simulink model "calibration_sensors"  (R2026a)
settings: Solver=VariableStepAuto  StopTime=inf
StopFcn:
  | coefficients = out.coefficients;
  | sensor_low = out.sensor_low;
  | sensor_high = out.sensor_high;
  | 
  | save('sensor_calibration.mat', ...
  |      'coefficients', ...
  |      'sensor_low', ...
  |      'sensor_high');
(part 1 of 3)
settings Model: Creator=user  LastModifiedBy=jinyu

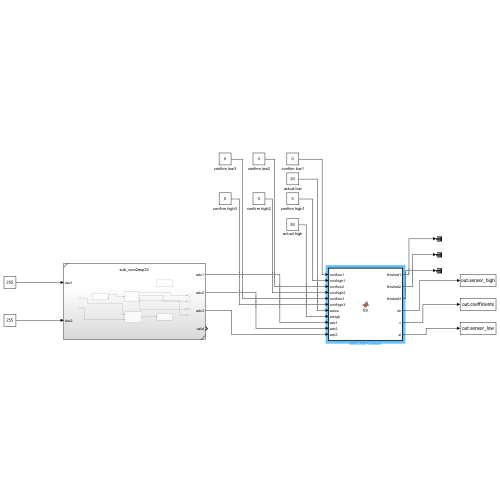
[thumbnail: Simulink's stored preview of the top-level diagram]
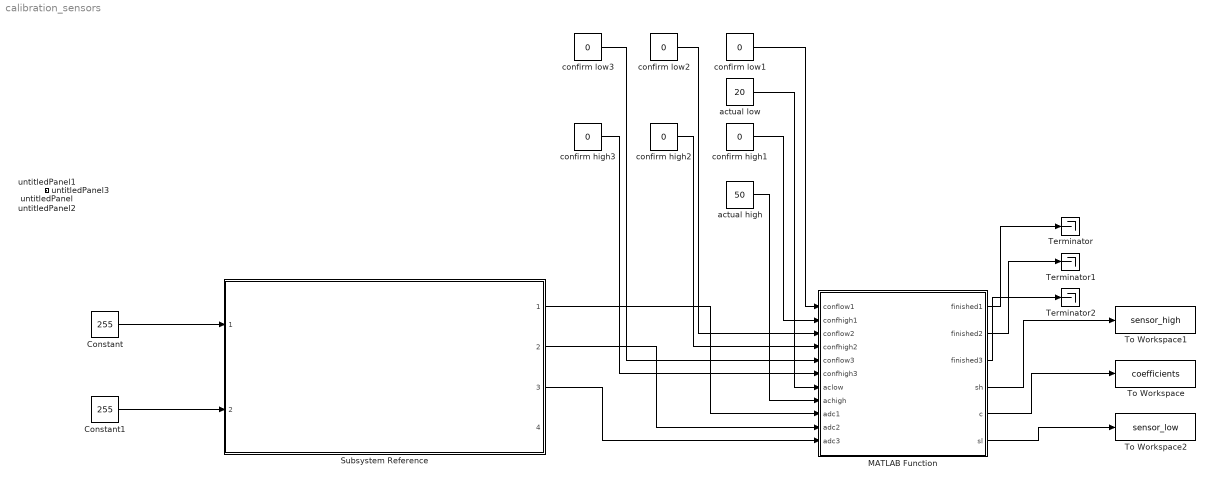
== system calibration_sensors ==
  Constant : Constant  Value=255
  Constant1 : Constant  Value=255
  MATLAB Function : MATLAB Function  TreatAsAtomicUnit=on
  Subsystem Reference : Subsystem  ReferencedSubsystem=sub_com2esp32
  Terminator : Terminator
  Terminator1 : Terminator
  Terminator2 : Terminator
  To Workspace : ToWorkspace  VariableName=coefficients  SampleTime=-1
      settings: MaxDataPoints=1
  To Workspace1 : ToWorkspace  VariableName=sensor_high  SampleTime=-1
      settings: MaxDataPoints=1
  To Workspace2 : ToWorkspace  VariableName=sensor_low  SampleTime=-1
      settings: MaxDataPoints=1
  actual high : Constant  Value=50
  actual low : Constant  Value=20
  confirm high1 : Constant  Value=0
  confirm high2 : Constant  Value=0
  confirm high3 : Constant  Value=0
  confirm low1 : Constant  Value=0
  confirm low2 : Constant  Value=0
  confirm low3 : Constant  Value=0
  untitledPanel : Subsystem  Tag=HiddenForWebPanel  IsWebBlockPanel=on
  untitledPanel1 : Subsystem  Tag=HiddenForWebPanel  IsWebBlockPanel=on
  untitledPanel2 : Subsystem  Tag=HiddenForWebPanel  IsWebBlockPanel=on
  untitledPanel3 : Subsystem  Tag=HiddenForWebPanel  IsWebBlockPanel=on
  wires:
  Constant/1 -> Subsystem Reference/1
  Constant1/1 -> Subsystem Reference/2
  Subsystem Reference/3 -> MATLAB Function/11(adc3)
  Subsystem Reference/1 -> MATLAB Function/9(adc1)
  Subsystem Reference/2 -> MATLAB Function/10(adc2)
  actual high/1 -> MATLAB Function/8(achigh)
  confirm high1/1 -> MATLAB Function/2(confhigh1)
  actual low/1 -> MATLAB Function/7(aclow)
  confirm low1/1 -> MATLAB Function/1(conflow1)
  MATLAB Function/5(c) -> To Workspace/1
  MATLAB Function/4(sh) -> To Workspace1/1
  MATLAB Function/6(sl) -> To Workspace2/1
  MATLAB Function/1(finished1) -> Terminator/1
  MATLAB Function/2(finished2) -> Terminator1/1
  confirm low2/1 -> MATLAB Function/3(conflow2)
  confirm high2/1 -> MATLAB Function/4(confhigh2)
  confirm low3/1 -> MATLAB Function/5(conflow3)
  confirm high3/1 -> MATLAB Function/6(confhigh3)
  MATLAB Function/3(finished3) -> Terminator2/1

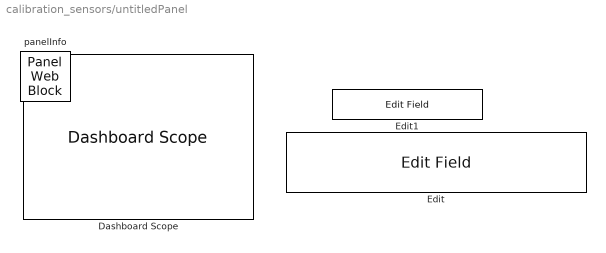
== system calibration_sensors/untitledPanel ==
  Dashboard Scope : DashboardScope  Tag=HiddenForWebPanel  PanelInfo="{\"height\":195,\"left\":22,\"panelId\":\"panelId-0a8f6d05-5e0e-4052-8464-4cdde78ccbfe\",\"top\":22,\"type\":\"panelChild\",\"version\":\"2019b\",\"width\":271,\"zIndex\":1500002}"  FontColor=[0.0, 0.0, 0.0]
  Edit : EditField  Tag=HiddenForWebPanel  PanelInfo="{\"height\":25,\"left\":322,\"panelId\":\"panelId-0a8f6d05-5e0e-4052-8464-4cdde78ccbfe\",\"top\":100,\"type\":\"panelChild\",\"version\":\"2019b\",\"width\":181,\"zIndex\":1500006}"  LabelPosition=Hide  ShowInitialText=on  Alignment=Center
  Edit1 : EditField  Tag=HiddenForWebPanel  PanelInfo="{\"height\":30,\"left\":327,\"panelId\":\"panelId-0a8f6d05-5e0e-4052-8464-4cdde78ccbfe\",\"top\":53,\"type\":\"panelChild\",\"version\":\"2019b\",\"width\":150,\"zIndex\":1500004}"  LabelPosition=Hide  ShowInitialText=on  Alignment=Center
  panelInfo : PanelWebBlock  Tag=HiddenForWebPanel  PanelInfo="{\"compacted\":false,\"height\":362,\"isActiveTab\":false,\"left\":183,\"name\":\"Panel\",\"panelId\":\"panelId-0a8f6d05-5e0e-4052-8464-4cdde78ccbfe\",\"popoutData\":{\"height\":495,\"left\":546,\"maximized\":false,\"top\":827,\"width\":618},\"popoutMode\":\"windowHidden\",\"tabIndex\":0,\"tabbedSetId\":\"tabbedSet4972758365\",\"top\":737,\"type\":\"panel\",\"version\":\"2019b\",\"visible\":false,\"width\":602,\"zIndex\":1500002}"  PanelSnapshot=<binary blob, 20028 chars, not shown>

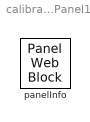
== system calibration_sensors/untitledPanel1 ==
  panelInfo : PanelWebBlock  Tag=HiddenForWebPanel  PanelInfo="{\"compacted\":false,\"height\":362,\"isActiveTab\":true,\"left\":183,\"name\":\"Panel1\",\"panelId\":\"panelId-b2ee2f41-7720-49f1-b51a-3062c351f597\",\"popoutData\":{\"height\":495,\"left\":546,\"maximized\":false,\"top\":827,\"width\":618},\"popoutMode\":\"windowHidden\",\"tabIndex\":1,\"tabbedSetId\":\"tabbedSet4972758365\",\"top\":737,\"type\":\"panel\",\"version\":\"2019b\",\"visible\":true,\"width\":602,\"zIndex\":1500004}"

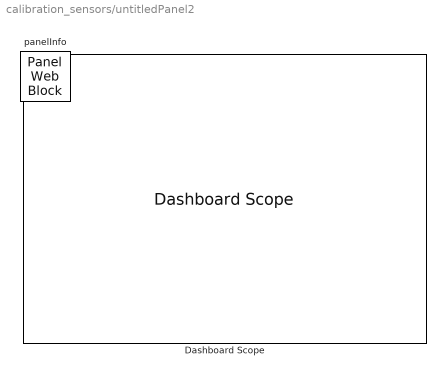
== system calibration_sensors/untitledPanel2 ==
  Dashboard Scope : DashboardScope  Tag=HiddenForWebPanel  PanelInfo="{\"height\":289,\"left\":18,\"panelId\":\"panelId-8ba459e9-7eb9-43d1-9a8b-2b7bff5a2d5c\",\"top\":18,\"type\":\"panelChild\",\"version\":\"2019b\",\"width\":403,\"zIndex\":1500002}"  FontColor=[0.0, 0.0, 0.0]
  panelInfo : PanelWebBlock  Tag=HiddenForWebPanel  PanelInfo="{\"compacted\":false,\"height\":329,\"isActiveTab\":true,\"left\":1320,\"name\":\"Panel2\",\"panelId\":\"panelId-8ba459e9-7eb9-43d1-9a8b-2b7bff5a2d5c\",\"popoutData\":{\"height\":440,\"left\":1683,\"maximized\":false,\"top\":822,\"width\":459},\"popoutMode\":\"windowHidden\",\"tabIndex\":0,\"tabbedSetId\":\"tabbedSet1724704130\",\"top\":710,\"type\":\"panel\",\"version\":\"2019b\",\"visible\":true,\"width\":443,\"zIndex\":1500006}"  PanelSnapshot=<binary blob, 75208 chars, not shown>
